simulink model "PV_Five_ModelWithGT"  (R2024b)
settings: Solver=VariableStepAuto  StartTime=0.0  StopTime=25  RelTol=1e-3
libraries: simulink x1
settings Model: Creator=86195  LastModifiedBy=86195

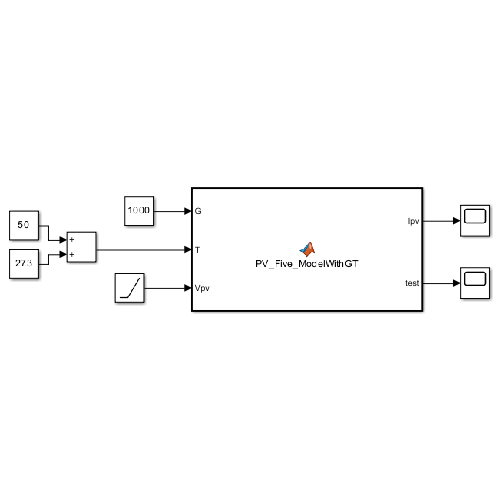
[thumbnail: Simulink's stored preview of the top-level diagram]
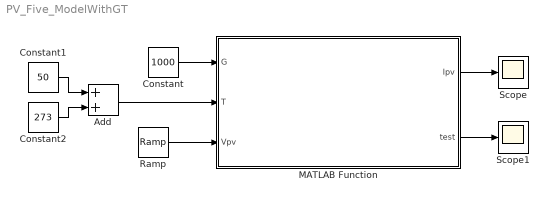
== system PV_Five_ModelWithGT ==
  Add : Sum
  Constant : Constant  Value=1000
  Constant1 : Constant  Value=50
  Constant2 : Constant  Value=273
  MATLAB Function : MATLAB Function  TreatAsAtomicUnit=on
  Ramp : simulink/Sources/Ramp  slope=1  start=0  InitialOutput=0
  Scope : Scope
  Scope1 : Scope
  wires:
  Constant/1 -> MATLAB Function/1(G)
  Constant1/1 -> Add/1
  Constant2/1 -> Add/2
  Add/1 -> MATLAB Function/2(T)
  Ramp/1 -> MATLAB Function/3(Vpv)
  MATLAB Function/1(Ipv) -> Scope/1
  MATLAB Function/2(test) -> Scope1/1

== matlab function PV_Five_ModelWithGT/MATLAB Function ==
  data: G input; Ipv output; T input; Vpv input; test output
function [Ipv, test] = PV_Five_ModelWithGT(G, T, Vpv)
    %% 光伏电池考虑温度、光照的五参数模型搭建
    
    %% 常数量
    k = 1.38e-23;      % 玻尔兹曼常数
    q = 1.60e-19;      % 单位电荷量
    Eg = 1.12;         % 硅材料带隙能量
    
    %% 已知参数
    G0 = 1000;         % 光照强度
    T0 = 25 + 273;     % 光伏电池温度
    A0 = 0.97359;      % 二极管的品质因数
    Iph0 = 3.8;        % 光生电流
    Is0 = 2.4515e-10;  % 二极管反向饱和电流
    Ns = 36;           % 光伏组件串联光伏单体数量
    Rp0 = 161.0752;    % 并联电阻
    Rs0 = 0.38659 / Ns;% 串联电阻
    Ki = 0.00065;      % 短路电流温度系数
    
    %% 初始化
    Ipv = zeros(size(Vpv));  % 初始化
    
    %% 公式计算
    Iph = (G / G0) * (Iph0 + Ki * (T - T0));
    A = A0;
    Is = Is0 * (T / T0)^3 * exp((q * Eg / (A * k)) * (1 / T0 - 1 / T));
    Rs = Rs0;
    Rp = Rp0 * (G0 / G);
    
    Vt = k * T / q;          % 光伏电池热电电压
    Vpv = Vpv / Ns;          % 计算每个串联光伏单体的电压
    Vd = Vpv + Ipv .* Rs;
    Id = Is * (exp(Vd ./ (A * Vt)) - 1);  % 注意跟理想模型不同，此处Vd不等于Vpv
    Ip = Vd ./ Rp;
    
    % 牛顿-拉夫逊法迭代计算
    for i = 1:10
        Ipv = Ipv - (Iph - Ipv - Id - Ip) ./ (-1 - (Id * Rs ./ (A * Vt)) - Rs / Rp);
    end
    
    test = exp((q * Eg / (A * k)) * (1 / T0 - 1 / T));
end
